simulink model "Plain_linmod"  (R2020b)
settings: Solver=VariableStepAuto  StartTime=0.0  StopTime=10.0  RelTol=1e-3
values from neighbouring files (symbols this model uses):
  X_init = [alpha_init;Omega_init(2);vA_init;Phi_init(2);Omega_init(3);beta_init;Omega_init(1);Phi_init(1); P_e_init(1);P_e_init(2);P_e_init(3);Phi_init(3)]    [SixDOFModel.m]
undefined symbols (not defined in the file or in its folder): Earth, nonlinear_6DOF, WGS84
libraries: aerolibtransform2 x1
settings Model: Creator=teteu  LastModifiedBy=teteu

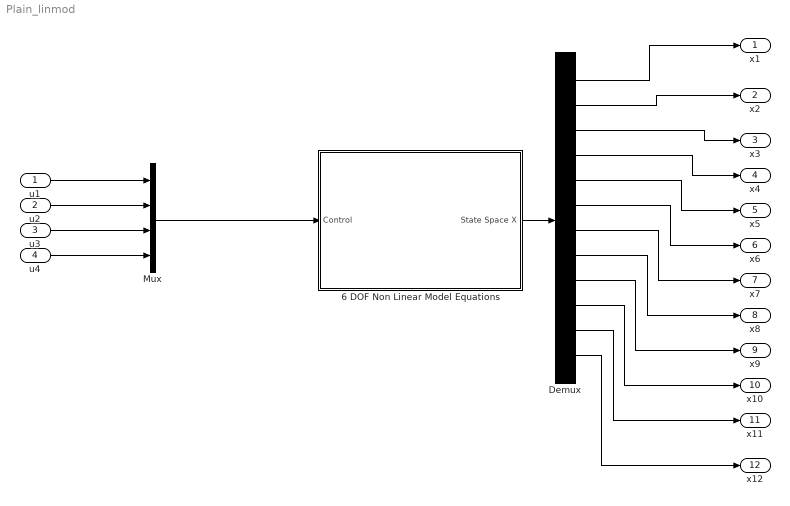
== system Plain_linmod ==
  u1 : Inport
  u2 : Inport  Port=2
  u3 : Inport  Port=3
  u4 : Inport  Port=4
  6 DOF Non Linear Model Equations : Subsystem
  Demux : Demux  Outputs=12
  Mux : Mux
  x1 : Outport
  x2 : Outport  Port=2
  x3 : Outport  Port=3
  x4 : Outport  Port=4
  x5 : Outport  Port=5
  x6 : Outport  Port=6
  x7 : Outport  Port=7
  x8 : Outport  Port=8
  x9 : Outport  Port=9
  x10 : Outport  Port=10
  x11 : Outport  Port=11
  x12 : Outport  Port=12
  wires:
  6 DOF Non Linear Model Equations/1(State Space X) -> Demux/1
  Demux/1 -> x1/1
  Demux/2 -> x2/1
  Demux/3 -> x3/1
  Demux/4 -> x4/1
  Demux/5 -> x5/1
  Demux/6 -> x6/1
  Demux/7 -> x7/1
  Demux/8 -> x8/1
  Demux/9 -> x9/1
  Demux/10 -> x10/1
  Demux/11 -> x11/1
  Demux/12 -> x12/1
  Mux/1 -> 6 DOF Non Linear Model Equations/1(Control)
  u1/1 -> Mux/1
  u2/1 -> Mux/2
  u3/1 -> Mux/3
  u4/1 -> Mux/4

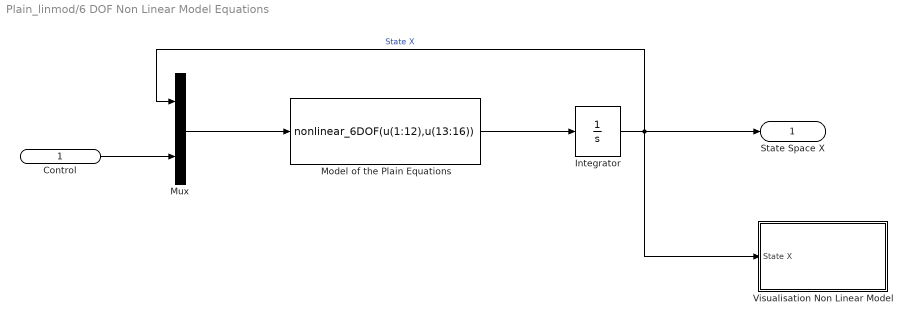
== system Plain_linmod/6 DOF Non Linear Model Equations ==
  Control : Inport
  Integrator : Integrator  InitialCondition=X_init
  Model of the Plain Equations : MATLABFcn  MATLABFcn=nonlinear_6DOF(u(1:12),u(13:16))
  Mux : Mux  Inputs=2
  Visualisation Non Linear Model : Subsystem
  State Space X : Outport
  wires:
  Model of the Plain Equations/1 -> Integrator/1
  Integrator/1 -> Visualisation Non Linear Model/1(State X), State Space X/1, Mux/1  "State X"
  Mux/1 -> Model of the Plain Equations/1
  Control/1 -> Mux/2

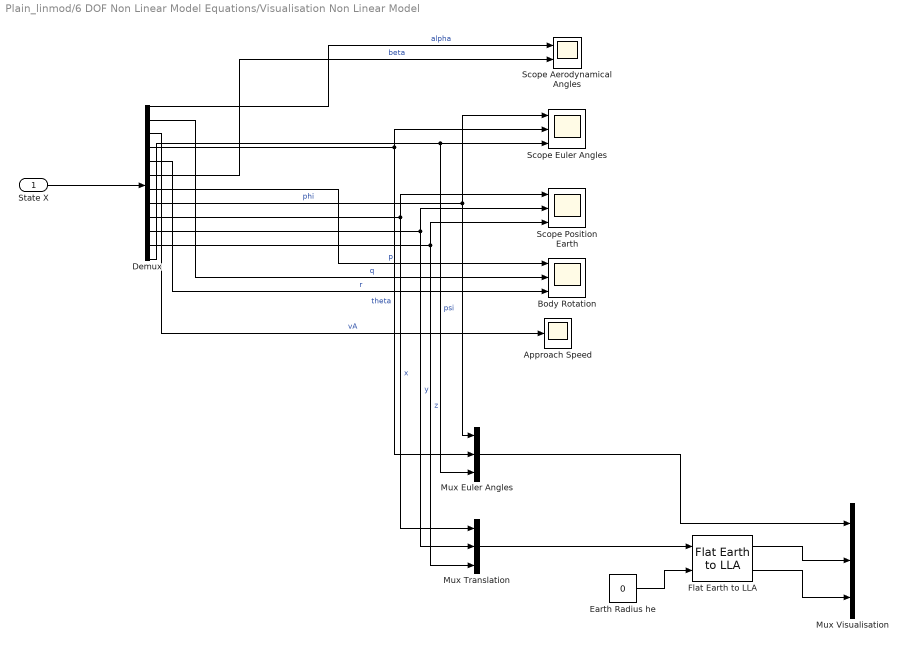
== system Plain_linmod/6 DOF Non Linear Model Equations/Visualisation Non Linear Model ==
  State X : Inport
  Approach Speed : Scope
  Body Rotation : Scope  NumInputPorts=3
  Demux : Demux  Outputs=12
  Earth Radius he : Constant  Value=0
  Flat Earth to LLA : aerolibtransform2/Flat Earth to LLA  units=Metric (MKS)  ptype=Earth (WGS84)  F=1/298.257223563  R=6378137  refPosPort=off  LL0=[0 10]  psi=0
  Mux Euler Angles : Mux  Inputs=3
  "Mux Translation " : Mux  Inputs=3
  Mux Visualisation : Mux  Inputs=3
  Scope Aerodynamical Angles : Scope  NumInputPorts=2
  Scope Euler Angles : Scope  NumInputPorts=3
  Scope Position Earth : Scope  NumInputPorts=3
  wires:
  Demux/4 -> Mux Euler Angles/2, Scope Euler Angles/2  "theta"
  Demux/10 -> Scope Position Earth/2, "Mux Translation "/2  "y"
  Demux/7 -> Body Rotation/1  "p"
  Demux/12 -> Scope Euler Angles/3, Mux Euler Angles/3  "psi"
  Demux/9 -> "Mux Translation "/1, Scope Position Earth/1  "x"
  Demux/8 -> Mux Euler Angles/1, Scope Euler Angles/1  "phi"
  Demux/6 -> Scope Aerodynamical Angles/2  "beta"
  Demux/3 -> Approach Speed/1  "vA"
  Demux/11 -> Scope Position Earth/3, "Mux Translation "/3  "z"
  Demux/1 -> Scope Aerodynamical Angles/1  "alpha"
  Demux/2 -> Body Rotation/2  "q"
  Demux/5 -> Body Rotation/3  "r"
  State X/1 -> Demux/1
  Flat Earth to LLA/1 -> Mux Visualisation/2
  Flat Earth to LLA/2 -> Mux Visualisation/3
  Earth Radius he/1 -> Flat Earth to LLA/2
  Mux Euler Angles/1 -> Mux Visualisation/1
  "Mux Translation "/1 -> Flat Earth to LLA/1
